simulink model "DCDC3_CL"  (R2024a)
settings: Solver=VariableStepAuto  StartTime=0.0  StopTime=Tsim_outLoop  FixedStep=Tstep  RelTol=1e-3
values from neighbouring files (symbols this model uses):
  deadtimesw = 2.8e-6    (= 2.8e-06)    [DCDC_param.m]
  ILmax = 10    [DCDC_param.m]
  Rload = VoutNom/IoutNom    (= 16.6666666667)    [DCDC_param.m]
  Tsw = 1/fsw    (= 0.0001)    [DCDC_param.m]    (also in adcpwm_setup.m)
  VinNom = 30    [DCDC_param.m]
  VoutNom = 50    [DCDC_param.m]
undefined symbols (not defined in the file or in its folder): den_aaf, DiscIntNeverNeededParam, kaw_i, kaw_v, ki_i, ki_v, kp_i, kp_v, kpf_i, kpf_v, num_aaf, Tstep, VLlim, zden_pf_i, zden_pf_v, znum_pf_i, znum_pf_v
libraries: simulink x30, nesl_utility x20, fl_lib x19, spsTriangleGeneratorLib x18, ee_lib x7
(part 2 of 2)

== system DCDC3_CL/innerLoop_currentControl1/PWM with Dead Time1 ==
  DC : Inport
  Compare To Zero1 : simulink/Logic and Bit Operations/Compare To Zero  relop=>=  OutDataTypeStr=boolean
  Compare To Zero2 : simulink/Logic and Bit Operations/Compare To Zero  relop=>=  OutDataTypeStr=boolean
  Data Type Conversion : DataTypeConversion  SaturateOnIntegerOverflow=off  RndMeth=Floor
  Data Type Conversion1 : DataTypeConversion  SaturateOnIntegerOverflow=off  RndMeth=Floor
  Fcn : Fcn  Expr=1-u(1)
  Fcn1 : Fcn  Expr=(u(1)+1)/2
  Fcn2 : Fcn  Expr=(u(1)+1)/2
  Fcn3 : Fcn  Expr=1-u(1)
  MATLAB Function : MATLAB Function  TreatAsAtomicUnit=on
  Scope : Scope  NumInputPorts=2
  Scope5 : Scope  NumInputPorts=2
  Sum : Sum  Inputs=|+-
  Sum1 : Sum  Inputs=+-|
  Triangle Generator : spsTriangleGeneratorLib/Triangle Generator  Freq=fsw  Phase=0  Ts=Tstep
  Triangle Generator1 : spsTriangleGeneratorLib/Triangle Generator  Freq=fsw  Phase=-(deadtimesw/Tsw)*360  Ts=Tstep
  SH : Outport
  SL : Outport  Port=2
  wires:
  Data Type Conversion/1 -> Fcn/1, Scope/1, MATLAB Function/3("SL ")  "SL"
  Fcn/1 -> MATLAB Function/1("SH ")  "SH"
  MATLAB Function/2(SL) -> SL/1, Scope5/2
  MATLAB Function/1(SH) -> SH/1, Scope5/1
  DC/1 -> Sum1/1, Sum/1
  Triangle Generator/1 -> Fcn1/1
  Sum/1 -> Compare To Zero1/1
  Fcn1/1 -> Sum/2
  Compare To Zero1/1 -> Data Type Conversion/1
  Triangle Generator1/1 -> Fcn2/1  "delayed carrier"
  Sum1/1 -> Compare To Zero2/1
  Compare To Zero2/1 -> Data Type Conversion1/1
  Fcn2/1 -> Sum1/2
  Data Type Conversion1/1 -> Fcn3/1, Scope/2, MATLAB Function/4(SLd)  "SLd"
  Fcn3/1 -> MATLAB Function/2(SHd)  "SHd"

== system DCDC3_CL/innerLoop_currentControl10/PWM with Dead Time ==
  DC : Inport
  Compare To Zero1 : simulink/Logic and Bit Operations/Compare To Zero  relop=>=  OutDataTypeStr=boolean
  Data Type Conversion : DataTypeConversion  SaturateOnIntegerOverflow=off  RndMeth=Floor
  Fcn : Fcn  Expr=1-u(1)
  Fcn1 : Fcn  Expr=(u(1)+1)/2
  MATLAB Function : MATLAB Function  TreatAsAtomicUnit=on
  Scope5 : Scope  NumInputPorts=2
  Sum : Sum  Inputs=|+-
  Transport Delay : TransportDelay  DelayTime=deadtimesw  InitialOutput=1
  Transport Delay1 : TransportDelay  DelayTime=deadtimesw  InitialOutput=1
  Triangle Generator : spsTriangleGeneratorLib/Triangle Generator  Freq=fsw  Phase=0  Ts=Tstep
  SH : Outport
  SL : Outport  Port=2
  wires:
  Transport Delay/1 -> MATLAB Function/2(SHd)
  Data Type Conversion/1 -> Transport Delay1/1, MATLAB Function/3("SL "), Fcn/1
  Fcn/1 -> MATLAB Function/1("SH "), Transport Delay/1
  MATLAB Function/2(SL) -> SL/1, Scope5/2
  Transport Delay1/1 -> MATLAB Function/4(SLd)
  MATLAB Function/1(SH) -> SH/1, Scope5/1
  DC/1 -> Sum/1
  Triangle Generator/1 -> Fcn1/1
  Sum/1 -> Compare To Zero1/1
  Fcn1/1 -> Sum/2
  Compare To Zero1/1 -> Data Type Conversion/1

== system DCDC3_CL/innerLoop_currentControl11/PWM with Dead Time ==
  DC : Inport
  Compare To Zero1 : simulink/Logic and Bit Operations/Compare To Zero  relop=>=  OutDataTypeStr=boolean
  Data Type Conversion : DataTypeConversion  SaturateOnIntegerOverflow=off  RndMeth=Floor
  Fcn : Fcn  Expr=1-u(1)
  Fcn1 : Fcn  Expr=(u(1)+1)/2
  MATLAB Function : MATLAB Function  TreatAsAtomicUnit=on
  Scope5 : Scope  NumInputPorts=2
  Sum : Sum  Inputs=|+-
  Transport Delay : TransportDelay  DelayTime=deadtimesw  InitialOutput=1
  Transport Delay1 : TransportDelay  DelayTime=deadtimesw  InitialOutput=1
  Triangle Generator : spsTriangleGeneratorLib/Triangle Generator  Freq=fsw  Phase=120  Ts=Tstep
  SH : Outport
  SL : Outport  Port=2
  wires:
  Transport Delay/1 -> MATLAB Function/2(SHd)
  Data Type Conversion/1 -> Transport Delay1/1, MATLAB Function/3("SL "), Fcn/1
  Fcn/1 -> MATLAB Function/1("SH "), Transport Delay/1
  MATLAB Function/2(SL) -> SL/1, Scope5/2
  Transport Delay1/1 -> MATLAB Function/4(SLd)
  MATLAB Function/1(SH) -> SH/1, Scope5/1
  DC/1 -> Sum/1
  Triangle Generator/1 -> Fcn1/1
  Sum/1 -> Compare To Zero1/1
  Fcn1/1 -> Sum/2
  Compare To Zero1/1 -> Data Type Conversion/1

== system DCDC3_CL/innerLoop_currentControl12/PWM with Dead Time ==
  DC : Inport
  Compare To Zero1 : simulink/Logic and Bit Operations/Compare To Zero  relop=>=  OutDataTypeStr=boolean
  Data Type Conversion : DataTypeConversion  SaturateOnIntegerOverflow=off  RndMeth=Floor
  Fcn : Fcn  Expr=1-u(1)
  Fcn1 : Fcn  Expr=(u(1)+1)/2
  MATLAB Function : MATLAB Function  TreatAsAtomicUnit=on
  Scope5 : Scope  NumInputPorts=2
  Sum : Sum  Inputs=|+-
  Transport Delay : TransportDelay  DelayTime=deadtimesw  InitialOutput=1
  Transport Delay1 : TransportDelay  DelayTime=deadtimesw  InitialOutput=1
  Triangle Generator : spsTriangleGeneratorLib/Triangle Generator  Freq=fsw  Phase=240  Ts=Tstep
  SH : Outport
  SL : Outport  Port=2
  wires:
  Transport Delay/1 -> MATLAB Function/2(SHd)
  Data Type Conversion/1 -> Transport Delay1/1, MATLAB Function/3("SL "), Fcn/1
  Fcn/1 -> MATLAB Function/1("SH "), Transport Delay/1
  MATLAB Function/2(SL) -> SL/1, Scope5/2
  Transport Delay1/1 -> MATLAB Function/4(SLd)
  MATLAB Function/1(SH) -> SH/1, Scope5/1
  DC/1 -> Sum/1
  Triangle Generator/1 -> Fcn1/1
  Sum/1 -> Compare To Zero1/1
  Fcn1/1 -> Sum/2
  Compare To Zero1/1 -> Data Type Conversion/1

== system DCDC3_CL/innerLoop_currentControl2/PWM with Dead Time2 ==
  DC : Inport
  Compare To Zero1 : simulink/Logic and Bit Operations/Compare To Zero  relop=>=  OutDataTypeStr=boolean
  Compare To Zero2 : simulink/Logic and Bit Operations/Compare To Zero  relop=>=  OutDataTypeStr=boolean
  Data Type Conversion : DataTypeConversion  SaturateOnIntegerOverflow=off  RndMeth=Floor
  Data Type Conversion1 : DataTypeConversion  SaturateOnIntegerOverflow=off  RndMeth=Floor
  Fcn : Fcn  Expr=1-u(1)
  Fcn1 : Fcn  Expr=(u(1)+1)/2
  Fcn2 : Fcn  Expr=(u(1)+1)/2
  Fcn3 : Fcn  Expr=1-u(1)
  MATLAB Function : MATLAB Function  TreatAsAtomicUnit=on
  Scope : Scope  NumInputPorts=2
  Scope5 : Scope  NumInputPorts=2
  Sum : Sum  Inputs=|+-
  Sum1 : Sum  Inputs=+-|
  Triangle Generator : spsTriangleGeneratorLib/Triangle Generator  Freq=fsw  Phase=120  Ts=Tstep
  Triangle Generator1 : spsTriangleGeneratorLib/Triangle Generator  Freq=fsw  Phase=120-(deadtimesw/Tsw)*360  Ts=Tstep
  SH : Outport
  SL : Outport  Port=2
  wires:
  Data Type Conversion/1 -> Fcn/1, Scope/1, MATLAB Function/3("SL ")  "SL"
  Fcn/1 -> MATLAB Function/1("SH ")  "SH"
  MATLAB Function/2(SL) -> SL/1, Scope5/2
  MATLAB Function/1(SH) -> SH/1, Scope5/1
  DC/1 -> Sum1/1, Sum/1
  Triangle Generator/1 -> Fcn1/1
  Sum/1 -> Compare To Zero1/1
  Fcn1/1 -> Sum/2
  Compare To Zero1/1 -> Data Type Conversion/1
  Triangle Generator1/1 -> Fcn2/1  "delayed carrier"
  Sum1/1 -> Compare To Zero2/1
  Compare To Zero2/1 -> Data Type Conversion1/1
  Fcn2/1 -> Sum1/2
  Data Type Conversion1/1 -> Fcn3/1, Scope/2, MATLAB Function/4(SLd)  "SLd"
  Fcn3/1 -> MATLAB Function/2(SHd)  "SHd"

== system DCDC3_CL/innerLoop_currentControl3/PWM with Dead Time3 ==
  DC : Inport
  Compare To Zero1 : simulink/Logic and Bit Operations/Compare To Zero  relop=>=  OutDataTypeStr=boolean
  Compare To Zero2 : simulink/Logic and Bit Operations/Compare To Zero  relop=>=  OutDataTypeStr=boolean
  Data Type Conversion : DataTypeConversion  SaturateOnIntegerOverflow=off  RndMeth=Floor
  Data Type Conversion1 : DataTypeConversion  SaturateOnIntegerOverflow=off  RndMeth=Floor
  Fcn : Fcn  Expr=1-u(1)
  Fcn1 : Fcn  Expr=(u(1)+1)/2
  Fcn2 : Fcn  Expr=(u(1)+1)/2
  Fcn3 : Fcn  Expr=1-u(1)
  MATLAB Function : MATLAB Function  TreatAsAtomicUnit=on
  Scope : Scope  NumInputPorts=2
  Scope5 : Scope  NumInputPorts=2
  Sum : Sum  Inputs=|+-
  Sum1 : Sum  Inputs=+-|
  Triangle Generator : spsTriangleGeneratorLib/Triangle Generator  Freq=fsw  Phase=240  Ts=Tstep
  Triangle Generator1 : spsTriangleGeneratorLib/Triangle Generator  Freq=fsw  Phase=240-(deadtimesw/Tsw)*360  Ts=Tstep
  SH : Outport
  SL : Outport  Port=2
  wires:
  Data Type Conversion/1 -> Fcn/1, Scope/1, MATLAB Function/3("SL ")  "SL"
  Fcn/1 -> MATLAB Function/1("SH ")  "SH"
  MATLAB Function/2(SL) -> SL/1, Scope5/2
  MATLAB Function/1(SH) -> SH/1, Scope5/1
  DC/1 -> Sum1/1, Sum/1
  Triangle Generator/1 -> Fcn1/1
  Sum/1 -> Compare To Zero1/1
  Fcn1/1 -> Sum/2
  Compare To Zero1/1 -> Data Type Conversion/1
  Triangle Generator1/1 -> Fcn2/1  "delayed carrier"
  Sum1/1 -> Compare To Zero2/1
  Compare To Zero2/1 -> Data Type Conversion1/1
  Fcn2/1 -> Sum1/2
  Data Type Conversion1/1 -> Fcn3/1, Scope/2, MATLAB Function/4(SLd)  "SLd"
  Fcn3/1 -> MATLAB Function/2(SHd)  "SHd"

== system DCDC3_CL/innerLoop_currentControl4/PWM with Dead Time ==
  DC : Inport
  Compare To Zero1 : simulink/Logic and Bit Operations/Compare To Zero  relop=>=  OutDataTypeStr=boolean
  Data Type Conversion : DataTypeConversion  SaturateOnIntegerOverflow=off  RndMeth=Floor
  Fcn : Fcn  Expr=1-u(1)
  Fcn1 : Fcn  Expr=(u(1)+1)/2
  MATLAB Function : MATLAB Function  TreatAsAtomicUnit=on
  Scope5 : Scope  NumInputPorts=2
  Sum : Sum  Inputs=|+-
  Transport Delay : TransportDelay  DelayTime=deadtimesw  InitialOutput=1
  Transport Delay1 : TransportDelay  DelayTime=deadtimesw  InitialOutput=1
  Triangle Generator : spsTriangleGeneratorLib/Triangle Generator  Freq=fsw  Phase=0  Ts=Tstep
  SH : Outport
  SL : Outport  Port=2
  wires:
  Transport Delay/1 -> MATLAB Function/2(SHd)
  Data Type Conversion/1 -> Transport Delay1/1, MATLAB Function/3("SL "), Fcn/1
  Fcn/1 -> MATLAB Function/1("SH "), Transport Delay/1
  MATLAB Function/2(SL) -> SL/1, Scope5/2
  Transport Delay1/1 -> MATLAB Function/4(SLd)
  MATLAB Function/1(SH) -> SH/1, Scope5/1
  DC/1 -> Sum/1
  Triangle Generator/1 -> Fcn1/1
  Sum/1 -> Compare To Zero1/1
  Fcn1/1 -> Sum/2
  Compare To Zero1/1 -> Data Type Conversion/1

== system DCDC3_CL/innerLoop_currentControl5/PWM with Dead Time ==
  DC : Inport
  Compare To Zero1 : simulink/Logic and Bit Operations/Compare To Zero  relop=>=  OutDataTypeStr=boolean
  Data Type Conversion : DataTypeConversion  SaturateOnIntegerOverflow=off  RndMeth=Floor
  Fcn : Fcn  Expr=1-u(1)
  Fcn1 : Fcn  Expr=(u(1)+1)/2
  MATLAB Function : MATLAB Function  TreatAsAtomicUnit=on
  Scope5 : Scope  NumInputPorts=2
  Sum : Sum  Inputs=|+-
  Transport Delay : TransportDelay  DelayTime=deadtimesw  InitialOutput=1
  Transport Delay1 : TransportDelay  DelayTime=deadtimesw  InitialOutput=1
  Triangle Generator : spsTriangleGeneratorLib/Triangle Generator  Freq=fsw  Phase=120  Ts=Tstep
  SH : Outport
  SL : Outport  Port=2
  wires:
  Transport Delay/1 -> MATLAB Function/2(SHd)
  Data Type Conversion/1 -> Transport Delay1/1, MATLAB Function/3("SL "), Fcn/1
  Fcn/1 -> MATLAB Function/1("SH "), Transport Delay/1
  MATLAB Function/2(SL) -> SL/1, Scope5/2
  Transport Delay1/1 -> MATLAB Function/4(SLd)
  MATLAB Function/1(SH) -> SH/1, Scope5/1
  DC/1 -> Sum/1
  Triangle Generator/1 -> Fcn1/1
  Sum/1 -> Compare To Zero1/1
  Fcn1/1 -> Sum/2
  Compare To Zero1/1 -> Data Type Conversion/1

== system DCDC3_CL/innerLoop_currentControl6/PWM with Dead Time ==
  DC : Inport
  Compare To Zero1 : simulink/Logic and Bit Operations/Compare To Zero  relop=>=  OutDataTypeStr=boolean
  Data Type Conversion : DataTypeConversion  SaturateOnIntegerOverflow=off  RndMeth=Floor
  Fcn : Fcn  Expr=1-u(1)
  Fcn1 : Fcn  Expr=(u(1)+1)/2
  MATLAB Function : MATLAB Function  TreatAsAtomicUnit=on
  Scope5 : Scope  NumInputPorts=2
  Sum : Sum  Inputs=|+-
  Transport Delay : TransportDelay  DelayTime=deadtimesw  InitialOutput=1
  Transport Delay1 : TransportDelay  DelayTime=deadtimesw  InitialOutput=1
  Triangle Generator : spsTriangleGeneratorLib/Triangle Generator  Freq=fsw  Phase=240  Ts=Tstep
  SH : Outport
  SL : Outport  Port=2
  wires:
  Transport Delay/1 -> MATLAB Function/2(SHd)
  Data Type Conversion/1 -> Transport Delay1/1, MATLAB Function/3("SL "), Fcn/1
  Fcn/1 -> MATLAB Function/1("SH "), Transport Delay/1
  MATLAB Function/2(SL) -> SL/1, Scope5/2
  Transport Delay1/1 -> MATLAB Function/4(SLd)
  MATLAB Function/1(SH) -> SH/1, Scope5/1
  DC/1 -> Sum/1
  Triangle Generator/1 -> Fcn1/1
  Sum/1 -> Compare To Zero1/1
  Fcn1/1 -> Sum/2
  Compare To Zero1/1 -> Data Type Conversion/1

== system DCDC3_CL/innerLoop_currentControl7/PWM with Dead Time1 ==
  DC : Inport
  Compare To Zero1 : simulink/Logic and Bit Operations/Compare To Zero  relop=>=  OutDataTypeStr=boolean
  Compare To Zero2 : simulink/Logic and Bit Operations/Compare To Zero  relop=>=  OutDataTypeStr=boolean
  Data Type Conversion : DataTypeConversion  SaturateOnIntegerOverflow=off  RndMeth=Floor
  Data Type Conversion1 : DataTypeConversion  SaturateOnIntegerOverflow=off  RndMeth=Floor
  Fcn : Fcn  Expr=1-u(1)
  Fcn1 : Fcn  Expr=(u(1)+1)/2
  Fcn2 : Fcn  Expr=(u(1)+1)/2
  Fcn3 : Fcn  Expr=1-u(1)
  MATLAB Function : MATLAB Function  TreatAsAtomicUnit=on
  Scope : Scope  NumInputPorts=2
  Scope5 : Scope  NumInputPorts=2
  Sum : Sum  Inputs=|+-
  Sum1 : Sum  Inputs=+-|
  Triangle Generator : spsTriangleGeneratorLib/Triangle Generator  Freq=fsw  Phase=0  Ts=Tstep
  Triangle Generator1 : spsTriangleGeneratorLib/Triangle Generator  Freq=fsw  Phase=-(deadtimesw/Tsw)*360  Ts=Tstep
  SH : Outport
  SL : Outport  Port=2
  wires:
  Data Type Conversion/1 -> Fcn/1, Scope/1, MATLAB Function/3("SL ")  "SL"
  Fcn/1 -> MATLAB Function/1("SH ")  "SH"
  MATLAB Function/2(SL) -> SL/1, Scope5/2
  MATLAB Function/1(SH) -> SH/1, Scope5/1
  DC/1 -> Sum1/1, Sum/1
  Triangle Generator/1 -> Fcn1/1
  Sum/1 -> Compare To Zero1/1
  Fcn1/1 -> Sum/2
  Compare To Zero1/1 -> Data Type Conversion/1
  Triangle Generator1/1 -> Fcn2/1  "delayed carrier"
  Sum1/1 -> Compare To Zero2/1
  Compare To Zero2/1 -> Data Type Conversion1/1
  Fcn2/1 -> Sum1/2
  Data Type Conversion1/1 -> Fcn3/1, Scope/2, MATLAB Function/4(SLd)  "SLd"
  Fcn3/1 -> MATLAB Function/2(SHd)  "SHd"

== system DCDC3_CL/innerLoop_currentControl8/PWM with Dead Time2 ==
  DC : Inport
  Compare To Zero1 : simulink/Logic and Bit Operations/Compare To Zero  relop=>=  OutDataTypeStr=boolean
  Compare To Zero2 : simulink/Logic and Bit Operations/Compare To Zero  relop=>=  OutDataTypeStr=boolean
  Data Type Conversion : DataTypeConversion  SaturateOnIntegerOverflow=off  RndMeth=Floor
  Data Type Conversion1 : DataTypeConversion  SaturateOnIntegerOverflow=off  RndMeth=Floor
  Fcn : Fcn  Expr=1-u(1)
  Fcn1 : Fcn  Expr=(u(1)+1)/2
  Fcn2 : Fcn  Expr=(u(1)+1)/2
  Fcn3 : Fcn  Expr=1-u(1)
  MATLAB Function : MATLAB Function  TreatAsAtomicUnit=on
  Scope : Scope  NumInputPorts=2
  Scope5 : Scope  NumInputPorts=2
  Sum : Sum  Inputs=|+-
  Sum1 : Sum  Inputs=+-|
  Triangle Generator : spsTriangleGeneratorLib/Triangle Generator  Freq=fsw  Phase=120  Ts=Tstep
  Triangle Generator1 : spsTriangleGeneratorLib/Triangle Generator  Freq=fsw  Phase=120-(deadtimesw/Tsw)*360  Ts=Tstep
  SH : Outport
  SL : Outport  Port=2
  wires:
  Data Type Conversion/1 -> Fcn/1, Scope/1, MATLAB Function/3("SL ")  "SL"
  Fcn/1 -> MATLAB Function/1("SH ")  "SH"
  MATLAB Function/2(SL) -> SL/1, Scope5/2
  MATLAB Function/1(SH) -> SH/1, Scope5/1
  DC/1 -> Sum1/1, Sum/1
  Triangle Generator/1 -> Fcn1/1
  Sum/1 -> Compare To Zero1/1
  Fcn1/1 -> Sum/2
  Compare To Zero1/1 -> Data Type Conversion/1
  Triangle Generator1/1 -> Fcn2/1  "delayed carrier"
  Sum1/1 -> Compare To Zero2/1
  Compare To Zero2/1 -> Data Type Conversion1/1
  Fcn2/1 -> Sum1/2
  Data Type Conversion1/1 -> Fcn3/1, Scope/2, MATLAB Function/4(SLd)  "SLd"
  Fcn3/1 -> MATLAB Function/2(SHd)  "SHd"

== system DCDC3_CL/innerLoop_currentControl9/PWM with Dead Time3 ==
  DC : Inport
  Compare To Zero1 : simulink/Logic and Bit Operations/Compare To Zero  relop=>=  OutDataTypeStr=boolean
  Compare To Zero2 : simulink/Logic and Bit Operations/Compare To Zero  relop=>=  OutDataTypeStr=boolean
  Data Type Conversion : DataTypeConversion  SaturateOnIntegerOverflow=off  RndMeth=Floor
  Data Type Conversion1 : DataTypeConversion  SaturateOnIntegerOverflow=off  RndMeth=Floor
  Fcn : Fcn  Expr=1-u(1)
  Fcn1 : Fcn  Expr=(u(1)+1)/2
  Fcn2 : Fcn  Expr=(u(1)+1)/2
  Fcn3 : Fcn  Expr=1-u(1)
  MATLAB Function : MATLAB Function  TreatAsAtomicUnit=on
  Scope : Scope  NumInputPorts=2
  Scope5 : Scope  NumInputPorts=2
  Sum : Sum  Inputs=|+-
  Sum1 : Sum  Inputs=+-|
  Triangle Generator : spsTriangleGeneratorLib/Triangle Generator  Freq=fsw  Phase=240  Ts=Tstep
  Triangle Generator1 : spsTriangleGeneratorLib/Triangle Generator  Freq=fsw  Phase=240-(deadtimesw/Tsw)*360  Ts=Tstep
  SH : Outport
  SL : Outport  Port=2
  wires:
  Data Type Conversion/1 -> Fcn/1, Scope/1, MATLAB Function/3("SL ")  "SL"
  Fcn/1 -> MATLAB Function/1("SH ")  "SH"
  MATLAB Function/2(SL) -> SL/1, Scope5/2
  MATLAB Function/1(SH) -> SH/1, Scope5/1
  DC/1 -> Sum1/1, Sum/1
  Triangle Generator/1 -> Fcn1/1
  Sum/1 -> Compare To Zero1/1
  Fcn1/1 -> Sum/2
  Compare To Zero1/1 -> Data Type Conversion/1
  Triangle Generator1/1 -> Fcn2/1  "delayed carrier"
  Sum1/1 -> Compare To Zero2/1
  Compare To Zero2/1 -> Data Type Conversion1/1
  Fcn2/1 -> Sum1/2
  Data Type Conversion1/1 -> Fcn3/1, Scope/2, MATLAB Function/4(SLd)  "SLd"
  Fcn3/1 -> MATLAB Function/2(SHd)  "SHd"

== matlab function DCDC3_CL/innerLoop_currentControl4/PWM with Dead Time/MATLAB Function ==
  data: SH input; SHd input; SH output; SL output; SL input; SLd input
function [SH,SL] = fcn(SH,SHd,SL,SLd)

if SHd + SH > 1
    SH = 1;
else
    SH = 0;
end

if SLd + SL > 1
    SL = 1;
else
    SL = 0;
end

== matlab function DCDC3_CL/innerLoop_currentControl4/VL2duty ==
  data: VLref input; D output; Vin_fb input; Vout_fb input
function D = fcn(VLref,Vin_fb,Vout_fb)

D = min([1 max([0 1 + (VLref - Vin_fb)/Vout_fb])]);

== matlab function DCDC3_CL/innerLoop_currentControl5/PWM with Dead Time/MATLAB Function ==
  data: SH input; SHd input; SH output; SL output; SL input; SLd input
function [SH,SL] = fcn(SH,SHd,SL,SLd)

if SHd + SH > 1
    SH = 1;
else
    SH = 0;
end

if SLd + SL > 1
    SL = 1;
else
    SL = 0;
end

== matlab function DCDC3_CL/innerLoop_currentControl5/VL2duty ==
  data: VLref input; D output; Vin_fb input; Vout_fb input
function D = fcn(VLref,Vin_fb,Vout_fb)

D = min([1 max([0 1 + (VLref - Vin_fb)/Vout_fb])]);

== matlab function DCDC3_CL/innerLoop_currentControl6/PWM with Dead Time/MATLAB Function ==
  data: SH input; SHd input; SH output; SL output; SL input; SLd input
function [SH,SL] = fcn(SH,SHd,SL,SLd)

if SHd + SH > 1
    SH = 1;
else
    SH = 0;
end

if SLd + SL > 1
    SL = 1;
else
    SL = 0;
end

== matlab function DCDC3_CL/innerLoop_currentControl6/VL2duty ==
  data: VLref input; D output; Vin_fb input; Vout_fb input
function D = fcn(VLref,Vin_fb,Vout_fb)

D = min([1 max([0 1 + (VLref - Vin_fb)/Vout_fb])]);

== matlab function DCDC3_CL/innerLoop_currentControl3/PWM with Dead Time3/MATLAB Function ==
  data: SH input; SHd input; SH output; SL output; SL input; SLd input
function [SH,SL] = fcn(SH,SHd,SL,SLd)

if SHd + SH > 1
    SH = 1;
else
    SH = 0;
end

if SLd + SL > 1
    SL = 1;
else
    SL = 0;
end

== matlab function DCDC3_CL/innerLoop_currentControl1/VL2duty ==
  data: VLref input; D output; Vin_fb input; Vout_fb input
function D = fcn(VLref,Vin_fb,Vout_fb)

D = min([1 max([0 1 + (VLref - Vin_fb)/Vout_fb])]);

== matlab function DCDC3_CL/Iout2IL3 ==
  data: K_Iout_IL output; ILref input; IoutRef input; VoutRef input; Vin input; ILref output; RserL parameter
function [K_Iout_IL,ILref] = fcn(ILref,IoutRef,VoutRef,Vin,RserL)

if VoutRef < Vin
    VoutRef = Vin;
end
K_Iout_IL = (Vin - RserL*ILref) / VoutRef;
ILref = IoutRef / K_Iout_IL;

== matlab function DCDC3_CL/innerLoop_currentControl10/PWM with Dead Time/MATLAB Function ==
  data: SH input; SHd input; SH output; SL output; SL input; SLd input
function [SH,SL] = fcn(SH,SHd,SL,SLd)

if SHd + SH > 1
    SH = 1;
else
    SH = 0;
end

if SLd + SL > 1
    SL = 1;
else
    SL = 0;
end

== matlab function DCDC3_CL/innerLoop_currentControl10/VL2duty ==
  data: VLref input; D output; Vin_fb input; Vout_fb input
function D = fcn(VLref,Vin_fb,Vout_fb)

D = min([1 max([0 1 + (VLref - Vin_fb)/Vout_fb])]);

== matlab function DCDC3_CL/innerLoop_currentControl11/PWM with Dead Time/MATLAB Function ==
  data: SH input; SHd input; SH output; SL output; SL input; SLd input
function [SH,SL] = fcn(SH,SHd,SL,SLd)

if SHd + SH > 1
    SH = 1;
else
    SH = 0;
end

if SLd + SL > 1
    SL = 1;
else
    SL = 0;
end

== matlab function DCDC3_CL/innerLoop_currentControl11/VL2duty ==
  data: VLref input; D output; Vin_fb input; Vout_fb input
function D = fcn(VLref,Vin_fb,Vout_fb)

D = min([1 max([0 1 + (VLref - Vin_fb)/Vout_fb])]);

== matlab function DCDC3_CL/innerLoop_currentControl12/PWM with Dead Time/MATLAB Function ==
  data: SH input; SHd input; SH output; SL output; SL input; SLd input
function [SH,SL] = fcn(SH,SHd,SL,SLd)

if SHd + SH > 1
    SH = 1;
else
    SH = 0;
end

if SLd + SL > 1
    SL = 1;
else
    SL = 0;
end

== matlab function DCDC3_CL/innerLoop_currentControl12/VL2duty ==
  data: VLref input; D output; Vin_fb input; Vout_fb input
function D = fcn(VLref,Vin_fb,Vout_fb)

D = min([1 max([0 1 + (VLref - Vin_fb)/Vout_fb])]);

== matlab function DCDC3_CL/innerLoop_currentControl7/PWM with Dead Time1/MATLAB Function ==
  data: SH input; SHd input; SH output; SL output; SL input; SLd input
function [SH,SL] = fcn(SH,SHd,SL,SLd)

if SHd + SH > 1
    SH = 1;
else
    SH = 0;
end

if SLd + SL > 1
    SL = 1;
else
    SL = 0;
end

== matlab function DCDC3_CL/innerLoop_currentControl7/VL2duty ==
  data: VLref input; D output; Vin_fb input; Vout_fb input
function D = fcn(VLref,Vin_fb,Vout_fb)

D = min([1 max([0 1 + (VLref - Vin_fb)/Vout_fb])]);

== matlab function DCDC3_CL/innerLoop_currentControl2/PWM with Dead Time2/MATLAB Function ==
  data: SH input; SHd input; SH output; SL output; SL input; SLd input
function [SH,SL] = fcn(SH,SHd,SL,SLd)

if SHd + SH > 1
    SH = 1;
else
    SH = 0;
end

if SLd + SL > 1
    SL = 1;
else
    SL = 0;
end

== matlab function DCDC3_CL/innerLoop_currentControl8/PWM with Dead Time2/MATLAB Function ==
  data: SH input; SHd input; SH output; SL output; SL input; SLd input
function [SH,SL] = fcn(SH,SHd,SL,SLd)

if SHd + SH > 1
    SH = 1;
else
    SH = 0;
end

if SLd + SL > 1
    SL = 1;
else
    SL = 0;
end

== matlab function DCDC3_CL/innerLoop_currentControl8/VL2duty ==
  data: VLref input; D output; Vin_fb input; Vout_fb input
function D = fcn(VLref,Vin_fb,Vout_fb)

D = min([1 max([0 1 + (VLref - Vin_fb)/Vout_fb])]);

== matlab function DCDC3_CL/innerLoop_currentControl9/PWM with Dead Time3/MATLAB Function ==
  data: SH input; SHd input; SH output; SL output; SL input; SLd input
function [SH,SL] = fcn(SH,SHd,SL,SLd)

if SHd + SH > 1
    SH = 1;
else
    SH = 0;
end

if SLd + SL > 1
    SL = 1;
else
    SL = 0;
end

== matlab function DCDC3_CL/innerLoop_currentControl9/VL2duty ==
  data: VLref input; D output; Vin_fb input; Vout_fb input
function D = fcn(VLref,Vin_fb,Vout_fb)

D = min([1 max([0 1 + (VLref - Vin_fb)/Vout_fb])]);

== matlab function DCDC3_CL/Iout2IL ==
  data: K_Iout_IL output; ILref input; IoutRef input; VoutRef input; Vin input; ILref output; RserL parameter
function [K_Iout_IL,ILref] = fcn(ILref,IoutRef,VoutRef,Vin,RserL)

if VoutRef < Vin
    VoutRef = Vin;
end
K_Iout_IL = (Vin - RserL*ILref) / VoutRef;
ILref = IoutRef / K_Iout_IL;

== matlab function DCDC3_CL/innerLoop_currentControl1/PWM with Dead Time1/MATLAB Function ==
  data: SH input; SHd input; SH output; SL output; SL input; SLd input
function [SH,SL] = fcn(SH,SHd,SL,SLd)

if SHd + SH > 1
    SH = 1;
else
    SH = 0;
end

if SLd + SL > 1
    SL = 1;
else
    SL = 0;
end

== matlab function DCDC3_CL/innerLoop_currentControl2/VL2duty ==
  data: VLref input; D output; Vin_fb input; Vout_fb input
function D = fcn(VLref,Vin_fb,Vout_fb)

D = min([1 max([0 1 + (VLref - Vin_fb)/Vout_fb])]);

== matlab function DCDC3_CL/Iout2IL1 ==
  data: K_Iout_IL output; ILref input; IoutRef input; VoutRef input; Vin input; ILref output; RserL parameter
function [K_Iout_IL,ILref] = fcn(ILref,IoutRef,VoutRef,Vin,RserL)

if VoutRef < Vin
    VoutRef = Vin;
end
K_Iout_IL = (Vin - RserL*ILref) / VoutRef;
ILref = IoutRef / K_Iout_IL;

== matlab function DCDC3_CL/innerLoop_currentControl3/VL2duty ==
  data: VLref input; D output; Vin_fb input; Vout_fb input
function D = fcn(VLref,Vin_fb,Vout_fb)

D = min([1 max([0 1 + (VLref - Vin_fb)/Vout_fb])]);

== matlab function DCDC3_CL/Iout2IL2 ==
  data: K_Iout_IL output; ILref input; IoutRef input; VoutRef input; Vin input; ILref output; RserL parameter
function [K_Iout_IL,ILref] = fcn(ILref,IoutRef,VoutRef,Vin,RserL)

if VoutRef < Vin
    VoutRef = Vin;
end
K_Iout_IL = (Vin - RserL*ILref) / VoutRef;
ILref = IoutRef / K_Iout_IL;
